simulink model "Michaels_CVModel_fast8"  (R2020a)
settings: Solver=ode23  StartTime=0.0  StopTime=30  RelTol=1e-2  EnableMultiTasking=on
model workspace (MAT data in the model file):
  Eao = 1.88
  Eesla = 0.58
  Eeslvf = 5.2
  Eesra = 0.63
  Eesrvf = 1.75
  Emaxspt = 48.75
  Epa = 0.15
  Epu = 0.04
  Esa = 0.37
  Esv = 0.013
  Evc = 0.03
  GpLV = 0
  GpRR = 11
  GpRV = 0
  GpRsa = 0
  GpV0 = 0
  GsLV = 0.007
  GsRR = 11
  GsRV = 0.022
  GsRsa = -0.05
  GsV0 = 31
  Ka = 4.4
  Lao = 0.0022
  Lav = 0.000354
  Lmt = 7.697e-05
  Lpa = 7.697e-05
  Lpv = 0.0001043
  Ltc = 8.009e-05
  P0la = 0.5
  P0lvf = 0.98
  P0pcd = 0.5
  P0ra = 0.5
  P0rvf = 0.91
  P0spt = 0.46
  PV : AO (value not decoded)
  PVao = [327.9; 100.9]
  Rao = 0.28
  Rav = 0.02
  Rla2pu = 0.5
  Rmt = 0.01
  Rpa = 0.12
  Rpa_Vals = 0.12
  Rpu = 0.006
  Rpv = 0.02
  Rra = 0.012
  Rsa = 0.74
  Rsv = 0.12
  Rtc = 0.01
  Tc = 1
  Tsys0 = 0.6
  V0la = 30
  V0lvf = 45
  V0pcd = 200
  V0ra = 25
  V0rvf = 50
  V0spt = 10
  Vdla = 15
  Vdlvf = 16
  Vdra = 15
  Vdrvf = 40
  Vdspt = 10
  Vlv0 = 100
  Vperi = 51
  Vrv0 = 105
  Vuao = 260.8
  Vupa = 91
  Vupu = 132
  Vusa = 287.4
  Vusv = 1976.1
  Vuvc = 136.17
  amin = -2
  artBrLVcontConti = []
  artBrLVcontDigi = [0 0 0 0 0 0 0 0 0 0 0 0 ... (240 elements, 1x240)]
  artBrRRConti = []
  artBrRRDigi = [0 0 0 0 0 0 0 0 0 0 1.57142857143 3.14285714286 ... (240 elements, 1x240)]
  artBrRVcontConti = []
  artBrRVcontDigi = [0 0 0 0 0 0 0 0 0 0 0 0 ... (240 elements, 1x240)]
  artBrRsaConti = []
  artBrRsaDigi = [0 0 0 0 0 0 0 0 0 0 0 0 ... (480 elements, 1x480)]
  artBrV0Conti = []
  artBrV0Digi = [0 0 0 0 0 0 0 0 0 0 0 0 ... (640 elements, 1x640)]
  atriumA = 1
  baroSampFreq = 16
  cP0la = 0.5
  cP0lvf = 0.98
  cP0ra = 0.5
  cP0rvf = 0.91
  cT = 1
  cVtotal = 5400
  clambdala = 0.13
  clambdalvf = 0.028
  clambdara = 0.13
  clambdarvf = 0.028
  deac = 0.0004
  ksys = 0.075
  lambdala = 0.065
  lambdalvf = 0.042
  lambdapcd = 0.005
  lambdara = 0.065
  lambdarvf = 0.028
  lambdaspt = 0.4
  pThor = 0
  params : object (value not decoded)
  sampleTime = 0.005
  svcPressureChange_MCS = 0
  svrMult = 1
  tStepOn = 1000000000
  t_baroOn = 1000000
  t_testBed_start = 1000000
  venk1 = 0.5
  venk2 = 0.5
symbols that are objects in the model workspace (value not decoded): PV
undefined symbols (not defined in the file): dfilt
libraries: simulink x85, fl_lib x39, nesl_utility x24, cstblocks x9, dspstat3 x9, dspobslib x5, SimscapeFluids_lib x5, sh_lib x1
(part 5 of 5)

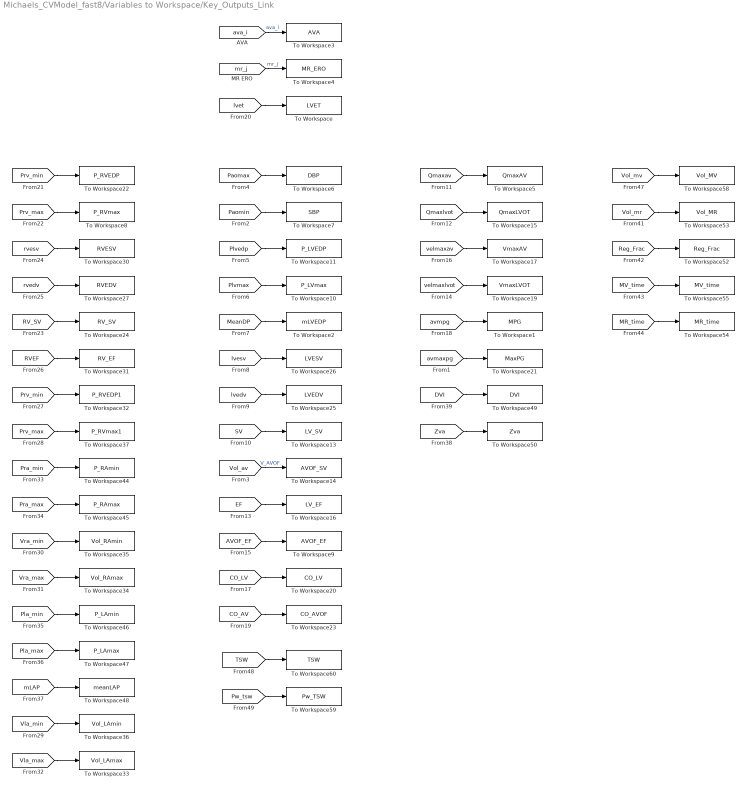
== system Michaels_CVModel_fast8/Variables to Workspace/Key_Outputs_Link ==
  To Workspace : ToWorkspace  VariableName=LVET  SampleTime=0.005
      settings: MaxDataPoints=1
  To Workspace1 : ToWorkspace  VariableName=MPG  SampleTime=0.01
      settings: MaxDataPoints=1
  To Workspace10 : ToWorkspace  VariableName=P_LVmax  SampleTime=0.01
      settings: MaxDataPoints=1
  To Workspace11 : ToWorkspace  VariableName=P_LVEDP  SampleTime=0.01
      settings: MaxDataPoints=1
  To Workspace13 : ToWorkspace  VariableName=LV_SV  SampleTime=0.01
      settings: MaxDataPoints=1
  To Workspace14 : ToWorkspace  VariableName=AVOF_SV  SampleTime=0.01
      settings: MaxDataPoints=1
  To Workspace15 : ToWorkspace  VariableName=QmaxLVOT  SampleTime=0.01
      settings: MaxDataPoints=1
  To Workspace16 : ToWorkspace  VariableName=LV_EF  SampleTime=0.01
      settings: MaxDataPoints=1
  To Workspace17 : ToWorkspace  VariableName=VmaxAV  SampleTime=0.01
      settings: MaxDataPoints=1
  To Workspace19 : ToWorkspace  VariableName=VmaxLVOT  SampleTime=0.01
      settings: MaxDataPoints=1
  To Workspace2 : ToWorkspace  VariableName=mLVEDP  SampleTime=0.01
      settings: MaxDataPoints=1
  To Workspace20 : ToWorkspace  VariableName=CO_LV  SampleTime=0.01
      settings: MaxDataPoints=1
  To Workspace21 : ToWorkspace  VariableName=MaxPG  SampleTime=0.01
      settings: MaxDataPoints=1
  To Workspace22 : ToWorkspace  VariableName=P_RVEDP  SampleTime=0.01
      settings: MaxDataPoints=1
  To Workspace23 : ToWorkspace  VariableName=CO_AVOF  SampleTime=0.01
      settings: MaxDataPoints=1
  To Workspace24 : ToWorkspace  VariableName=RV_SV  SampleTime=0.01
      settings: MaxDataPoints=1
  To Workspace25 : ToWorkspace  VariableName=LVEDV  SampleTime=0.01
      settings: MaxDataPoints=1
  To Workspace26 : ToWorkspace  VariableName=LVESV  SampleTime=0.01
      settings: MaxDataPoints=1
  To Workspace27 : ToWorkspace  VariableName=RVEDV  SampleTime=0.01
      settings: MaxDataPoints=1
  To Workspace3 : ToWorkspace  VariableName=AVA  SampleTime=0.005
      settings: MaxDataPoints=1
  To Workspace30 : ToWorkspace  VariableName=RVESV  SampleTime=0.01
      settings: MaxDataPoints=1
  To Workspace31 : ToWorkspace  VariableName=RV_EF  SampleTime=0.01
      settings: MaxDataPoints=1
  To Workspace32 : ToWorkspace  VariableName=P_RVEDP1  SampleTime=0.01
      settings: MaxDataPoints=1
  To Workspace33 : ToWorkspace  VariableName=Vol_LAmax  SampleTime=0.01
      settings: MaxDataPoints=1
  To Workspace34 : ToWorkspace  VariableName=Vol_RAmax  SampleTime=0.01
      settings: MaxDataPoints=1
  To Workspace35 : ToWorkspace  VariableName=Vol_RAmin  SampleTime=0.01
      settings: MaxDataPoints=1
  To Workspace36 : ToWorkspace  VariableName=Vol_LAmin  SampleTime=0.01
      settings: MaxDataPoints=1
  To Workspace37 : ToWorkspace  VariableName=P_RVmax1  SampleTime=0.01
      settings: MaxDataPoints=1
  To Workspace4 : ToWorkspace  VariableName=MR_ERO  SampleTime=0.005
      settings: MaxDataPoints=1
  To Workspace44 : ToWorkspace  VariableName=P_RAmin  SampleTime=0.01
      settings: MaxDataPoints=1
  To Workspace45 : ToWorkspace  VariableName=P_RAmax  SampleTime=0.01
      settings: MaxDataPoints=1
  To Workspace46 : ToWorkspace  VariableName=P_LAmin  SampleTime=0.01
      settings: MaxDataPoints=1
  To Workspace47 : ToWorkspace  VariableName=P_LAmax  SampleTime=0.01
      settings: MaxDataPoints=1
  To Workspace48 : ToWorkspace  VariableName=meanLAP  SampleTime=0.01
      settings: MaxDataPoints=1
  To Workspace49 : ToWorkspace  VariableName=DVI  SampleTime=0.01
      settings: MaxDataPoints=1
  To Workspace5 : ToWorkspace  VariableName=QmaxAV  SampleTime=0.01
      settings: MaxDataPoints=1
  To Workspace50 : ToWorkspace  VariableName=Zva  SampleTime=0.01
      settings: MaxDataPoints=1
  To Workspace52 : ToWorkspace  VariableName=Reg_Frac  SampleTime=0.01
      settings: MaxDataPoints=1
  To Workspace53 : ToWorkspace  VariableName=Vol_MR  SampleTime=0.01
      settings: MaxDataPoints=1
  To Workspace54 : ToWorkspace  VariableName=MR_time  SampleTime=0.01
      settings: MaxDataPoints=1
  To Workspace55 : ToWorkspace  VariableName=MV_time  SampleTime=0.01
      settings: MaxDataPoints=1
  To Workspace58 : ToWorkspace  VariableName=Vol_MV  SampleTime=0.01
      settings: MaxDataPoints=1
  To Workspace59 : ToWorkspace  VariableName=Pw_TSW  SampleTime=0.01
      settings: MaxDataPoints=1
  To Workspace6 : ToWorkspace  VariableName=DBP  SampleTime=0.01
      settings: MaxDataPoints=1
  To Workspace60 : ToWorkspace  VariableName=TSW  SampleTime=0.01
      settings: MaxDataPoints=1
  To Workspace7 : ToWorkspace  VariableName=SBP  SampleTime=0.01
      settings: MaxDataPoints=1
  To Workspace8 : ToWorkspace  VariableName=P_RVmax  SampleTime=0.01
      settings: MaxDataPoints=1
  To Workspace9 : ToWorkspace  VariableName=AVOF_EF  SampleTime=0.01
      settings: MaxDataPoints=1
  wires:
  [ava_i] -> To Workspace3/1  "ava_i"
  [mr_j] -> To Workspace4/1  "mr_j"
  [Paomax] -> To Workspace6/1
  [Paomin] -> To Workspace7/1
  [Plvedp] -> To Workspace11/1
  [Plvmax] -> To Workspace10/1
  [MeanDP] -> To Workspace2/1
  [lvedv] -> To Workspace25/1
  [lvesv] -> To Workspace26/1
  [SV] -> To Workspace13/1
  [Vol_av] -> To Workspace14/1  "V_AVOF"
  [Qmaxav] -> To Workspace5/1
  [Qmaxlvot] -> To Workspace15/1
  [EF] -> To Workspace16/1
  [velmaxlvot] -> To Workspace19/1
  [velmaxav] -> To Workspace17/1
  [avmpg] -> To Workspace1/1
  [avmaxpg] -> To Workspace21/1
  [CO_LV] -> To Workspace20/1
  [CO_AV] -> To Workspace23/1
  [lvet] -> To Workspace/1
  [rvesv] -> To Workspace30/1
  [rvedv] -> To Workspace27/1
  [Prv_max] -> To Workspace8/1
  [Prv_min] -> To Workspace22/1
  [RVEF] -> To Workspace31/1
  [RV_SV] -> To Workspace24/1
  [Prv_min] -> To Workspace32/1
  [Prv_max] -> To Workspace37/1
  [Vra_min] -> To Workspace35/1
  [Pra_min] -> To Workspace44/1
  [Pra_max] -> To Workspace45/1
  [Vra_max] -> To Workspace34/1
  [Vla_max] -> To Workspace33/1
  [Pla_max] -> To Workspace47/1
  [Pla_min] -> To Workspace46/1
  [Vla_min] -> To Workspace36/1
  [mLAP] -> To Workspace48/1
  [Zva] -> To Workspace50/1
  [DVI] -> To Workspace49/1
  [Vol_mr] -> To Workspace53/1
  [Reg_Frac] -> To Workspace52/1
  [MR_time] -> To Workspace54/1
  [MV_time] -> To Workspace55/1
  [Vol_mv] -> To Workspace58/1
  [Pw_tsw] -> To Workspace59/1
  [TSW] -> To Workspace60/1
  [AVOF_EF] -> To Workspace9/1

== system Michaels_CVModel_fast8/Variables to Workspace/Pressure ==
  From1 : From  Commented=on  GotoTag=Pthor2  TagVisibility=global
      settings: CloseFcn=tagdialog Close
  From44 : From  Commented=on  GotoTag=Prv  TagVisibility=global
      settings: CloseFcn=tagdialog Close
  From45 : From  Commented=on  GotoTag=Pla  TagVisibility=global
      settings: CloseFcn=tagdialog Close
  From46 : From  Commented=on  GotoTag=Pra  TagVisibility=global
      settings: CloseFcn=tagdialog Close
  From47 : From  Commented=on  GotoTag=Ppa  TagVisibility=global
      settings: CloseFcn=tagdialog Close
  From48 : From  Commented=on  GotoTag=Ppu  TagVisibility=global
      settings: CloseFcn=tagdialog Close
  From49 : From  Commented=on  GotoTag=Psa  TagVisibility=global
      settings: CloseFcn=tagdialog Close
  From50 : From  Commented=on  GotoTag=Psv  TagVisibility=global
      settings: CloseFcn=tagdialog Close
  From51 : From  Commented=on  GotoTag=Pao  TagVisibility=global
      settings: CloseFcn=tagdialog Close
  From52 : From  Commented=on  GotoTag=Pvc  TagVisibility=global
      settings: CloseFcn=tagdialog Close
  From53 : From  Commented=on  GotoTag=Pthor  TagVisibility=global
      settings: CloseFcn=tagdialog Close
  To Workspace1 : ToWorkspace  VariableName=P_LV  SampleTime=0.005
      settings: MaxDataPoints=201
  To Workspace10 : ToWorkspace  Commented=on  VariableName=P_THOR  SampleTime=0.005
  To Workspace11 : ToWorkspace  Commented=on  VariableName=P_VC  SampleTime=0.005
  To Workspace12 : ToWorkspace  Commented=on  VariableName=P_THOR2  SampleTime=0.005
  To Workspace13 : ToWorkspace  VariableName=P_LV2  SampleTime=0.005
      settings: MaxDataPoints=201
  To Workspace2 : ToWorkspace  Commented=on  VariableName=P_RV  SampleTime=0.005
  To Workspace3 : ToWorkspace  Commented=on  VariableName=P_LA  SampleTime=0.005
  To Workspace4 : ToWorkspace  Commented=on  VariableName=P_RA  SampleTime=0.005
  To Workspace5 : ToWorkspace  Commented=on  VariableName=P_SA  SampleTime=0.005
  To Workspace6 : ToWorkspace  Commented=on  VariableName=P_AO  SampleTime=0.005
  To Workspace7 : ToWorkspace  Commented=on  VariableName=P_SV  SampleTime=0.005
  To Workspace8 : ToWorkspace  Commented=on  VariableName=P_PA  SampleTime=0.005
  To Workspace9 : ToWorkspace  Commented=on  VariableName=P_PU  SampleTime=0.005
  wires:
  [Plv] -> To Workspace1/1  "P_LV"
  From44/1 -> To Workspace2/1  "P_RV"
  From45/1 -> To Workspace3/1  "P_LA"
  From46/1 -> To Workspace4/1  "P_RA"
  From49/1 -> To Workspace5/1  "P_SA"
  From51/1 -> To Workspace6/1  "P_AO"
  From50/1 -> To Workspace7/1  "P_SV"
  From47/1 -> To Workspace8/1  "P_PA"
  From48/1 -> To Workspace9/1  "P_PU"
  From53/1 -> To Workspace10/1  "P_THOR"
  From52/1 -> To Workspace11/1  "P_VC"
  From1/1 -> To Workspace12/1
  [PLV_SSc] -> To Workspace13/1

== system Michaels_CVModel_fast8/Variables to Workspace/Settings ==
  01Constant42 : Constant  Value=Eeslvf
  02Constant46 : Constant  Value=Eesrvf
  03Constant28 : Constant  Value=Eesla
  04Constant38 : Constant  Value=Eesra
  101Constant1 : Constant  Value=Eao
  101Constant2 : Constant  Value=Rao
  10Constant1 : Constant  Value=Vusa
  10Constant2 : Constant  Value=Rpu
  10Constant43 : Constant  Value=Vdlvf
  11Constant1 : Constant  Value=Vuao
  11Constant2 : Constant  Value=Lao
  11Constant41 : Constant  Value=V0lvf
  12Constant47 : Constant  Value=Vdrvf
  13Constant45 : Constant  Value=V0rvf
  14Constant29 : Constant  Value=Vdla
  15Constant27 : Constant  Value=V0la
  16Constant39 : Constant  Value=Vdra
  17Constant37 : Constant  Value=V0ra
  18Constant30 : Constant  Value=V0pcd
  20Constant34 : Constant  Value=lambdalvf
  21Constant35 : Constant  Value=lambdarvf
  22Constant32 : Constant  Value=lambdala
  23Constant33 : Constant  Value=lambdara
  24Constant36 : Constant  Value=lambdapcd
  5Constant44 : Constant  Value=P0lvf
  6Constant48 : Constant  Value=P0rvf
  7Constant31 : Constant  Value=P0la
  8Constant40 : Constant  Value=P0ra
  9Constant49 : Constant  Value=P0pcd
  Mux1 : Mux  Inputs=18
  Mux2 : Mux  Inputs=8
  Mux3 : Mux  Inputs=6
  Rla2pu : Constant  Value=Rla2pu
  Settings : Scope  Commented=on  NumInputPorts=2
  Settings1 : Scope  Commented=on
  wires:
  18Constant30/1 -> Mux1/18  "V0pcd"
  9Constant49/1 -> Mux1/17  "P0pcd"
  8Constant40/1 -> Mux1/16  "P0ra"
  16Constant39/1 -> Mux1/15  "Vdra"
  17Constant37/1 -> Mux1/14  "V0ra"
  04Constant38/1 -> Mux1/13  "Eesra"
  7Constant31/1 -> Mux1/12  "P0la"
  14Constant29/1 -> Mux1/11  "Vdla"
  15Constant27/1 -> Mux1/10  "V0la"
  03Constant28/1 -> Mux1/9  "Eesla"
  6Constant48/1 -> Mux1/8  "P0rvf"
  12Constant47/1 -> Mux1/7  "Vdrvf"
  13Constant45/1 -> Mux1/6  "V0rvf"
  02Constant46/1 -> Mux1/5  "Eesrvf"
  5Constant44/1 -> Mux1/4  "P0lvf"
  10Constant43/1 -> Mux1/3  "Vdlvf"
  11Constant41/1 -> Mux1/2  "V0lvf"
  01Constant42/1 -> Mux1/1  "Eeslvf"
  22Constant32/1 -> Mux2/1  "lambdala"
  23Constant33/1 -> Mux2/2  "lambdara"
  20Constant34/1 -> Mux2/3  "lambdalvf"
  21Constant35/1 -> Mux2/4  "lambdarvf"
  24Constant36/1 -> Mux2/5  "lambdapcd"
  Mux1/1 -> Settings/1
  Mux2/1 -> Settings/2
  [Rsa] -> Mux2/6  "xRsa"
  [Vusv] -> Mux2/7  "xVusv"
  Rla2pu/1 -> Mux2/8  "xRla2Pu"
  11Constant1/1 -> Mux3/2  "Vuao"
  101Constant1/1 -> Mux3/1  "Eesao"
  10Constant1/1 -> Mux3/3  "Vusa"
  101Constant2/1 -> Mux3/4  "Rao"
  11Constant2/1 -> Mux3/5  "Lao"
  10Constant2/1 -> Mux3/6  "Rpu"
  Mux3/1 -> Settings1/1

== system Michaels_CVModel_fast8/Variables to Workspace/Volume ==
  From1 : From  Commented=on  GotoTag=AVOF_Vol  TagVisibility=global
      settings: CloseFcn=tagdialog Close
  From54 : From  Commented=on  GotoTag=Vlv  TagVisibility=global
      settings: CloseFcn=tagdialog Close
  From55 : From  Commented=on  GotoTag=Vrv  TagVisibility=global
      settings: CloseFcn=tagdialog Close
  From56 : From  Commented=on  GotoTag=Vla  TagVisibility=global
      settings: CloseFcn=tagdialog Close
  From57 : From  Commented=on  GotoTag=Vra  TagVisibility=global
      settings: CloseFcn=tagdialog Close
  From58 : From  Commented=on  GotoTag=Vsv  TagVisibility=global
      settings: CloseFcn=tagdialog Close
  From59 : From  Commented=on  GotoTag=Vsa  TagVisibility=global
      settings: CloseFcn=tagdialog Close
  From60 : From  Commented=on  GotoTag=Vpa  TagVisibility=global
      settings: CloseFcn=tagdialog Close
  From61 : From  Commented=on  GotoTag=Vpu  TagVisibility=global
      settings: CloseFcn=tagdialog Close
  From62 : From  Commented=on  GotoTag=Vspt  TagVisibility=global
      settings: CloseFcn=tagdialog Close
  From63 : From  Commented=on  GotoTag=Vvc  TagVisibility=global
      settings: CloseFcn=tagdialog Close
  From64 : From  Commented=on  GotoTag=Vao  TagVisibility=global
      settings: CloseFcn=tagdialog Close
  To Workspace1 : ToWorkspace  Commented=on  VariableName=V_AV  SampleTime=0.005
      settings: MaxDataPoints=201
  To Workspace13 : ToWorkspace  VariableName=V_Total  SampleTime=0.005
  To Workspace14 : ToWorkspace  Commented=on  VariableName=V_VC  SampleTime=0.005
  To Workspace15 : ToWorkspace  Commented=on  VariableName=V_RV  SampleTime=0.005
  To Workspace16 : ToWorkspace  Commented=on  VariableName=V_LA  SampleTime=0.005
  To Workspace17 : ToWorkspace  Commented=on  VariableName=V_RA  SampleTime=0.005
  To Workspace18 : ToWorkspace  Commented=on  VariableName=V_SA  SampleTime=0.005
  To Workspace19 : ToWorkspace  Commented=on  VariableName=V_AO  SampleTime=0.005
  To Workspace2 : ToWorkspace  Commented=on  VariableName=V_LV  SampleTime=0.005
      settings: MaxDataPoints=201  Save2DSignal=2-D array (concatenate along first dimension)
  To Workspace20 : ToWorkspace  Commented=on  VariableName=V_SV  SampleTime=0.005
  To Workspace21 : ToWorkspace  Commented=on  VariableName=V_PA  SampleTime=0.005
  To Workspace23 : ToWorkspace  Commented=on  VariableName=V_spt  SampleTime=0.005
  To Workspace24 : ToWorkspace  Commented=on  VariableName=V_PU  SampleTime=0.005
  wires:
  From54/1 -> To Workspace2/1  "V_LV"
  From55/1 -> To Workspace15/1  "V_RV"
  From56/1 -> To Workspace16/1  "V_LA"
  From57/1 -> To Workspace17/1  "V_RA"
  From62/1 -> To Workspace23/1  "V_SPT"
  [Vtotal] -> To Workspace13/1  "V_Total"
  From63/1 -> To Workspace14/1  "V_VC"
  From59/1 -> To Workspace18/1  "V_SA"
  From64/1 -> To Workspace19/1  "V_AO"
  From58/1 -> To Workspace20/1  "V_SV"
  From60/1 -> To Workspace21/1  "V_PA"
  From61/1 -> To Workspace24/1  "V_PU"
  From1/1 -> To Workspace1/1  "V_AVOF"

== system Michaels_CVModel_fast8/ev/Activation - Atria ==
  note: Activation Functions - atria
  Action 1 - Sin Squared : Subsystem  TreatAsAtomicUnit=on
  Action 2 - cos Squared1 : Subsystem  TreatAsAtomicUnit=on
  Condition 1 : Subsystem
  Condition 2 : Subsystem
  Else - 0 : Subsystem  TreatAsAtomicUnit=on
  If : If  NumInputs=2  IfExpression=u1 == 1  ElseIfExpressions=u2 == 1
  Mux : Mux  Inputs=3
  Mux1 : Mux
  Mux2 : Mux  Commented=on  Inputs=2
  Scope2 : Scope  Commented=on
  ea : Merge  Inputs=3
  Out1 : Outport
  wires:
  Condition 1/1(Out1) -> If/1, Mux2/1
  Condition 2/1(Out1) -> If/2, Mux2/2
  If/3 -> Else - 0/Action
  Else - 0/1(Out1) -> ea/3
  [Tsh_a] -> Mux/2, Mux1/2
  [t] -> Mux/1, Mux1/1
  [Tr_A] -> Mux/3, Mux1/3
  Mux/1 -> Action 1 - Sin Squared/1(In1)
  If/1 -> Action 1 - Sin Squared/Action
  Mux1/1 -> Action 2 - cos Squared1/1(In1)
  If/2 -> Action 2 - cos Squared1/Action
  [TsysA] -> Mux1/4
  Action 1 - Sin Squared/1(Out1) -> ea/1
  Action 2 - cos Squared1/1(Out1) -> ea/2
  Mux2/1 -> Scope2/1
  ea/1 -> Out1/1

== system Michaels_CVModel_fast8/ev/Activation - Ventricle ==
  note: Activation Functions - Ventricle
  Action 1 - Sin Squared : Subsystem  TreatAsAtomicUnit=on
  Action 2 - cos Squared1 : Subsystem  TreatAsAtomicUnit=on
  Condition 1 : Subsystem
  Condition 2 : Subsystem
  Else - 0 : Subsystem  TreatAsAtomicUnit=on
  If : If  NumInputs=2  IfExpression=u1 == 1  ElseIfExpressions=u2 == 1
  Mux : Mux  Inputs=3
  Mux1 : Mux
  Mux2 : Mux  Commented=on  Inputs=2
  Scope2 : Scope  Commented=on
  ev : Merge  Inputs=3
  1 : Outport
  wires:
  Condition 1/1(Out1) -> If/1, Mux2/1
  Condition 2/1(Out1) -> If/2, Mux2/2
  If/3 -> Else - 0/Action
  Else - 0/1(Out1) -> ev/3
  [Tsh_v] -> Mux/2, Mux1/2
  [t] -> Mux/1, Mux1/1
  [Tr_V] -> Mux/3, Mux1/3
  Mux/1 -> Action 1 - Sin Squared/1(In1)
  If/1 -> Action 1 - Sin Squared/Action
  Mux1/1 -> Action 2 - cos Squared1/1(In1)
  If/2 -> Action 2 - cos Squared1/Action
  [TsysV] -> Mux1/4
  Action 1 - Sin Squared/1(Out1) -> ev/1
  Action 2 - cos Squared1/1(Out1) -> ev/2
  Mux2/1 -> Scope2/1
  ev/1 -> 1/1

== system Michaels_CVModel_fast8/ev/Activation - Ventricle_half ==
  note: Activation Functions - Ventricle
  Action 1 - Sin Squared : Subsystem  TreatAsAtomicUnit=on
  Action 2 - cos Squared1 : Subsystem  TreatAsAtomicUnit=on
  Condition 1 : Subsystem
  Condition 2 : Subsystem
  Else - 0 : Subsystem  TreatAsAtomicUnit=on
  If : If  NumInputs=2  IfExpression=u1 == 1  ElseIfExpressions=u2 == 1
  Mux : Mux  Inputs=3
  Mux1 : Mux
  Mux2 : Mux  Commented=on  Inputs=2
  Scope2 : Scope  Commented=on
  ev : Merge  Inputs=3
  evcos : Outport
  wires:
  Condition 1/1(Out1) -> If/1, Mux2/1
  Condition 2/1(Out1) -> If/2, Mux2/2
  If/3 -> Else - 0/Action
  Else - 0/1(Out1) -> ev/3
  [Tsh_v] -> Mux/2, Mux1/2
  [t] -> Mux/1, Mux1/1
  [Tr_V] -> Mux/3, Mux1/3
  Mux/1 -> Action 1 - Sin Squared/1(In1)
  If/1 -> Action 1 - Sin Squared/Action
  Mux1/1 -> Action 2 - cos Squared1/1(In1)
  If/2 -> Action 2 - cos Squared1/Action
  [TsysV] -> Mux1/4
  Action 1 - Sin Squared/1(Out1) -> ev/1
  Action 2 - cos Squared1/1(Out1) -> ev/2
  Mux2/1 -> Scope2/1
  ev/1 -> evcos/1

== system Michaels_CVModel_fast8/ev/Ev off-set ==
  note: Offset to reduce delay btw LV response to activation
  Inport : Inport
  Add : Sum  Inputs=+-
  Constant : Constant  Value=0.001
  Gain2 : Gain  Gain=1.001
  Saturation : Saturate  UpperLimit=inf  LowerLimit=0
  " " : Outport
  wires:
  Gain2/1 -> Add/1
  Add/1 -> Saturation/1
  Constant/1 -> Add/2
  Inport/1 -> Gain2/1
  Saturation/1 -> " "/1

== system Michaels_CVModel_fast8/Baroreflex/Baroreflex Heldt/avg filter ==
  Raw : Inport
  Buffer : Buffer  N=1.5*1/0.01  V=1.5*1/0.01-1
  Fcn : Fcn  Expr=(u(1)+u(2))/2
  MinMax : MinMax
  MinMax1 : MinMax  Function=max
  Mux : Mux  Inputs=2
  Mux1 : Mux  Commented=on
  SH 0.01 : ZeroOrderHold  SampleTime=0.01
  Scope : Scope  Commented=on
  Unbuffer : Unbuffer
  Unbuffer1 : Unbuffer
  Avg : Outport
  wires:
  Raw/1 -> SH 0.01/1, Mux1/4
  SH 0.01/1 -> Buffer/1
  Buffer/1 -> MinMax/1, MinMax1/1
  MinMax1/1 -> Unbuffer/1
  Mux/1 -> Fcn/1
  Unbuffer/1 -> Mux/2, Mux1/2
  MinMax/1 -> Unbuffer1/1
  Unbuffer1/1 -> Mux/1, Mux1/1
  Fcn/1 -> Avg/1, Mux1/3
  Mux1/1 -> Scope/1

== system Michaels_CVModel_fast8/Baroreflex/Baroreflex Heldt/sigmoid limit ==
  In1 : Inport
  Gain : Gain  Gain=1/18
  Gain1 : Gain  Gain=18
  Trigonometric Function : Trigonometry  Operator=atan
  Out1 : Outport
  wires:
  Gain/1 -> Trigonometric Function/1
  Trigonometric Function/1 -> Gain1/1
  In1/1 -> Gain/1
  Gain1/1 -> Out1/1

== system Michaels_CVModel_fast8/Baroreflex/Baroreflex Heldt cont/Filter ==
  Raw : Inport
  Buffer : Buffer  N=1.5*1/0.01  V=1.5*1/0.01-1
  Fcn : Fcn  Expr=(1*u(1)+1*u(2))/2
  MinMax : MinMax  Function=max
  MinMax1 : MinMax
  Mux : Mux  Inputs=2
  Mux1 : Mux
  SH 0.01 : ZeroOrderHold  SampleTime=0.01
  Scope : Scope  Commented=on
  Unbuffer : Unbuffer
  Unbuffer1 : Unbuffer
  Filtered : Outport
  wires:
  Raw/1 -> SH 0.01/1, Mux1/4
  SH 0.01/1 -> Buffer/1
  Buffer/1 -> MinMax/1, MinMax1/1
  MinMax1/1 -> Unbuffer/1
  Mux/1 -> Fcn/1
  Unbuffer/1 -> Mux/2, Mux1/2
  MinMax/1 -> Unbuffer1/1
  Unbuffer1/1 -> Mux/1, Mux1/1
  Fcn/1 -> Filtered/1, Mux1/3
  Mux1/1 -> Scope/1

== system Michaels_CVModel_fast8/Baroreflex/Baroreflex Heldt cont/sigmoid limit ==
  In1 : Inport
  Gain : Gain  Gain=1/18
  Gain1 : Gain  Gain=18
  Trigonometric Function : Trigonometry  Operator=atan
  Out1 : Outport
  wires:
  Gain/1 -> Trigonometric Function/1
  Trigonometric Function/1 -> Gain1/1
  In1/1 -> Gain/1
  Gain1/1 -> Out1/1

== system Michaels_CVModel_fast8/Graphs and Scopes/SW Scrap/Stroke Work Action ==
  In1 : Inport
  Inport2 : Inport  Port=2
  Action Port : ActionPort
  Integrator1 : Integrator  ExternalReset=rising
  Integrator2 : Integrator  ExternalReset=rising
  Integrator3 : Integrator  ExternalReset=rising
  Product : Product
  Scope : Scope  NumInputPorts=2
  Outport : Outport
  wires:
  Integrator1/1 -> Scope/1, Outport/1
  Product/1 -> Integrator1/1
  Inport2/1 -> Product/2, Scope/2, Integrator1/2
  In1/1 -> Product/1

== system Michaels_CVModel_fast8/Graphs and Scopes/SW Scrap/Stroke Work Action1 ==
  In1 : Inport
  Inport2 : Inport  Port=2
  Action Port : ActionPort
  Integrator2 : Integrator  ExternalReset=rising
  Integrator3 : Integrator  ExternalReset=rising
  Product : Product
  Scope : Scope  NumInputPorts=2
  Outport : Outport
  wires:
  In1/1 -> Product/1
  Inport2/1 -> Scope/2, Product/2
  Product/1 -> Scope/1, Outport/1

== system Michaels_CVModel_fast8/Graphs and Scopes/SW Scrap/Stroke Work Action2 ==
  In1 : Inport
  In2 : Inport  Port=2
  Inport2 : Inport  Port=3
  Action Port : ActionPort  InitializeStates=reset
  Integrator1 : Integrator  ExternalReset=either
  Product : Product
  Scope : Scope  NumInputPorts=2
  Outport : Outport
  wires:
  In1/1 -> Product/1
  Inport2/1 -> Product/2
  Product/1 -> Integrator1/1
  Integrator1/1 -> Outport/1, Scope/1
  In2/1 -> Integrator1/2

== system Michaels_CVModel_fast8/Graphs and Scopes/SW Scrap/Stroke Work Action3 ==
  In1 : Inport
  Inport2 : Inport  Port=2
  Action Port : ActionPort  InitializeStates=reset
  Integrator : Integrator  ExternalReset=either
  Product : Product
  Scope : Scope  NumInputPorts=2
  Outport : Outport
  wires:
  Product/1 -> Integrator/1
  Inport2/1 -> Product/2, Scope/2
  In1/1 -> Integrator/2, Product/1
  Integrator/1 -> Outport/1, Scope/1

== system Michaels_CVModel_fast8/Graphs and Scopes/SW Scrap/Stroke Work Action5 ==
  In1 : Inport
  Inport2 : Inport  Port=2
  Action Port : ActionPort
  Integrator1 : Integrator  ExternalReset=rising
  Product : Product
  Scope : Scope  NumInputPorts=2
  Outport : Outport
  wires:
  Integrator1/1 -> Scope/1, Outport/1
  Product/1 -> Integrator1/1
  Inport2/1 -> Integrator1/2, Product/2
  In1/1 -> Product/1

== system Michaels_CVModel_fast8/Graphs and Scopes/SW Scrap/Stroke Work Action6 ==
  In1 : Inport
  Inport2 : Inport  Port=2
  Action Port : ActionPort
  Integrator : Integrator  ExternalReset=rising
  Product : Product
  Scope : Scope  NumInputPorts=2
  Outport : Outport
  wires:
  Integrator/1 -> Scope/1, Outport/1
  In1/1 -> Integrator/2, Product/1
  Inport2/1 -> Scope/2, Product/2
  Product/1 -> Integrator/1

== system Michaels_CVModel_fast8/Graphs and Scopes/SW Scrap/Triggered Subsystem ==
  Outport : Inport
  Trigger : TriggerPort  VariantControl=(inherit)
  SW Q_AV1 : Outport  VectorParamsAs1DForOutWhenUnconnected=off
  wires:
  Outport/1 -> SW Q_AV1/1  "SW"

== system Michaels_CVModel_fast8/Graphs and Scopes/SW Scrap/Triggered Subsystem1 ==
  Outport : Inport
  Trigger : TriggerPort  VariantControl=(inherit)
  SW Q_AV1 : Outport  VectorParamsAs1DForOutWhenUnconnected=off
  wires:
  Outport/1 -> SW Q_AV1/1  "SW"

== system Michaels_CVModel_fast8/Graphs and Scopes/SW Scrap/Triggered Subsystem3 ==
  Outport : Inport
  Trigger : TriggerPort  VariantControl=(inherit)
  SW Q_AV1 : Outport  VectorParamsAs1DForOutWhenUnconnected=off
  wires:
  Outport/1 -> SW Q_AV1/1  "SW"

== system Michaels_CVModel_fast8/Stroke Work Calcs/Stroke Work Calc AVOF/Triggered Subsystem ==
  In1 : Inport
  In2 : Inport  Port=2
  Trigger : TriggerPort  TriggerType=falling  VariantControl=(inherit)
  Out1 : Outport  VectorParamsAs1DForOutWhenUnconnected=off
  Out2 : Outport  Port=2  VectorParamsAs1DForOutWhenUnconnected=off
  wires:
  In2/1 -> Out2/1  "SW"
  In1/1 -> Out1/1  "Energy"

== system Michaels_CVModel_fast8/Stroke Work Calcs/Stroke Work MR_Vol/Triggered Subsystem ==
  In1 : Inport
  In2 : Inport  Port=2
  Trigger : TriggerPort  TriggerType=falling  VariantControl=(inherit)
  Out1 : Outport  VectorParamsAs1DForOutWhenUnconnected=off
  Out2 : Outport  Port=2  VectorParamsAs1DForOutWhenUnconnected=off
  wires:
  In2/1 -> Out2/1  "SW"
  In1/1 -> Out1/1  "Energy"

== system Michaels_CVModel_fast8/Stroke Work Calcs/Stroke Work Q_AV/Stroke Work Action ==
  In1 : Inport
  In2 : Inport  Port=2
  Inport2 : Inport  Port=3
  Action Port : ActionPort  InitializeStates=reset  ActionPortLabel=if(u1 == 1)
  Integrator1 : Integrator  ExternalReset=rising
  Product : Product
  Scope : Scope  Commented=on  NumInputPorts=2
  Outport : Outport
  wires:
  In2/1 -> Integrator1/2
  In1/1 -> Product/1
  Inport2/1 -> Product/2, Scope/2
  Product/1 -> Integrator1/1
  Integrator1/1 -> Outport/1, Scope/1

== system Michaels_CVModel_fast8/Stroke Work Calcs/Stroke Work Q_AV/Triggered Subsystem1 ==
  Outport : Inport
  Trigger : TriggerPort  TriggerType=falling  VariantControl=(inherit)
  2a1 : simulink/Math Operations/MinMax Running Resettable  Description=2a  Function=max  vinit=0
  Pulse Generator3 : DiscretePulseGenerator  PulseType=Time based  Period=20  PhaseDelay=23.7
  SW Q_AV : Outport  VectorParamsAs1DForOutWhenUnconnected=off
  wires:
  Pulse Generator3/1 -> 2a1/2
  ? -> 2a1/1
  Outport/1 -> SW Q_AV/1  "SW"

== system Michaels_CVModel_fast8/Stroke Work Calcs/Stroke Work Q_MR/MR Stroke Work Action ==
  PLV : Inport
  QMR : Inport  Port=2
  MRreg : Inport  Port=3
  Action Port : ActionPort  InitializeStates=reset  ActionPortLabel=if(u1 == 1)
  Integrator1 : Integrator  ExternalReset=rising  ZeroCross=off
  Product : Product
  Outport : Outport
  wires:
  PLV/1 -> Product/1
  QMR/1 -> Product/2
  Product/1 -> Integrator1/1
  Integrator1/1 -> Outport/1
  MRreg/1 -> Integrator1/2

== system Michaels_CVModel_fast8/Stroke Work Calcs/Stroke Work Q_MR/Triggered Subsystem1 ==
  Inport : Inport
  Trigger : TriggerPort  TriggerType=falling  VariantControl=(inherit)
  RSW_ Q : Outport  VectorParamsAs1DForOutWhenUnconnected=off
  wires:
  Inport/1 -> RSW_ Q/1  "SW"

== system Michaels_CVModel_fast8/Stroke Work Calcs/Total Stroke Work LV/Triggered Subsystem ==
  In1 : Inport
  In2 : Inport  Port=2
  Trigger : TriggerPort  VariantControl=(inherit)
  Out1 : Outport  VectorParamsAs1DForOutWhenUnconnected=off
  Out2 : Outport  Port=2  VectorParamsAs1DForOutWhenUnconnected=off
  wires:
  In2/1 -> Out2/1  "SW"
  In1/1 -> Out1/1  "Energy"

== system Michaels_CVModel_fast8/ev/Activation - Atria/Action 1 - Sin Squared ==
  In1 : Inport
  Action Port : ActionPort  ActionPortLabel=if(u1 == 1)
  Demux : Demux  Outputs=3
  Gain : Gain  Gain=pi()
  Gain1 : Gain  Gain=2
  Math Function : Math  Operator=square  SignedPower=on  SaturateOnIntegerOverflow=on
  Product18 : Product  Inputs=*/  InputSameDT=on  RndMeth=Zero  SaturateOnIntegerOverflow=on  OutDataTypeStr=Inherit: Same as first input
  Sum3 : Sum  Inputs=+-  InputSameDT=on  SaturateOnIntegerOverflow=on  OutDataTypeStr=Inherit: Same as first input
  Trigonometric Function : Trigonometry
  Out1 : Outport
  wires:
  In1/1 -> Demux/1
  Demux/1 -> Sum3/1  "t"
  Demux/2 -> Sum3/2  "tsh_v"
  Sum3/1 -> Gain/1
  Gain/1 -> Product18/1
  Demux/3 -> Gain1/1
  Gain1/1 -> Product18/2
  Product18/1 -> Trigonometric Function/1
  Trigonometric Function/1 -> Math Function/1
  Math Function/1 -> Out1/1

== system Michaels_CVModel_fast8/ev/Activation - Atria/Action 2 - cos Squared1 ==
  In1 : Inport
  Action Port : ActionPort  ActionPortLabel=elseif(u2 == 1)
  Demux : Demux
  Gain : Gain  Gain=pi()
  Gain1 : Gain  Gain=2
  Math Function : Math  Operator=square  SignedPower=on  SaturateOnIntegerOverflow=on
  Product18 : Product  Inputs=*/  InputSameDT=on  RndMeth=Zero  SaturateOnIntegerOverflow=on  OutDataTypeStr=Inherit: Same as first input
  Sum1 : Sum  Inputs=+-  InputSameDT=on  SaturateOnIntegerOverflow=on  OutDataTypeStr=Inherit: Same as first input
  Sum3 : Sum  Inputs=+--  InputSameDT=on  SaturateOnIntegerOverflow=on  OutDataTypeStr=Inherit: Same as first input
  Trigonometric Function : Trigonometry  Operator=cos
  Out1 : Outport
  wires:
  In1/1 -> Demux/1
  Demux/1 -> Sum3/1  "t"
  Demux/2 -> Sum3/2  "tsh_v"
  Sum3/1 -> Gain/1
  Gain/1 -> Product18/1
  Gain1/1 -> Product18/2
  Product18/1 -> Trigonometric Function/1
  Trigonometric Function/1 -> Math Function/1
  Math Function/1 -> Out1/1
  Demux/3 -> Sum3/3, Sum1/2  "tr"
  Sum1/1 -> Gain1/1
  Demux/4 -> Sum1/1

== system Michaels_CVModel_fast8/ev/Activation - Atria/Condition 1 ==
  note: Condition 1 - Start of Systole
  Logical Operator : Logic  AllPortsSameDT=off  OutDataTypeStr=boolean
  Relational Operator : RelationalOperator  OutDataTypeStr=boolean  RndMeth=Nearest
  Relational Operator1 : RelationalOperator  Operator=<  OutDataTypeStr=boolean  RndMeth=Nearest
  Sum4 : Sum  InputSameDT=on  SaturateOnIntegerOverflow=on  OutDataTypeStr=Inherit: Same as first input
  Out1 : Outport
  wires:
  [t] -> Relational Operator/1
  [Tsh_a] -> Relational Operator/2
  [t] -> Relational Operator1/1
  [Tsh_a] -> Sum4/1
  [Tr_A] -> Sum4/2
  Sum4/1 -> Relational Operator1/2
  Relational Operator/1 -> Logical Operator/1
  Relational Operator1/1 -> Logical Operator/2
  Logical Operator/1 -> Out1/1

== system Michaels_CVModel_fast8/ev/Activation - Atria/Condition 2 ==
  note: Condition 2 - End of Systole
  Logical Operator1 : Logic  AllPortsSameDT=off  OutDataTypeStr=boolean
  Relational Operator2 : RelationalOperator  OutDataTypeStr=boolean  RndMeth=Nearest
  Relational Operator3 : RelationalOperator  Operator=<  OutDataTypeStr=boolean  RndMeth=Nearest
  Sum5 : Sum  InputSameDT=on  SaturateOnIntegerOverflow=on  OutDataTypeStr=Inherit: Same as first input
  Sum6 : Sum  InputSameDT=on  SaturateOnIntegerOverflow=on  OutDataTypeStr=Inherit: Same as first input
  Out1 : Outport
  wires:
  [t] -> Relational Operator2/1
  [t] -> Relational Operator3/1
  [Tsh_a] -> Sum5/1
  [Tr_A] -> Sum5/2
  Relational Operator2/1 -> Logical Operator1/1
  Relational Operator3/1 -> Logical Operator1/2
  Sum5/1 -> Relational Operator2/2
  [Tsh_a] -> Sum6/1
  [TsysA] -> Sum6/2
  Sum6/1 -> Relational Operator3/2
  Logical Operator1/1 -> Out1/1

== system Michaels_CVModel_fast8/ev/Activation - Atria/Else - 0 ==
  Action Port : ActionPort  ActionPortLabel=else
  venk3 : Constant  Value=0
  Out1 : Outport
  wires:
  venk3/1 -> Out1/1

== system Michaels_CVModel_fast8/ev/Activation - Ventricle/Action 1 - Sin Squared ==
  In1 : Inport
  Action Port : ActionPort  ActionPortLabel=if(u1 == 1)
  Demux : Demux  Outputs=3
  Gain : Gain  Gain=pi()
  Gain1 : Gain  Gain=2
  Math Function : Math  Operator=square  SignedPower=on  SaturateOnIntegerOverflow=on
  Product18 : Product  Inputs=*/  InputSameDT=on  RndMeth=Zero  SaturateOnIntegerOverflow=on  OutDataTypeStr=Inherit: Same as first input
  Sum3 : Sum  Inputs=+-  InputSameDT=on  SaturateOnIntegerOverflow=on  OutDataTypeStr=Inherit: Same as first input
  Trigonometric Function : Trigonometry
  Out1 : Outport
  wires:
  In1/1 -> Demux/1
  Demux/1 -> Sum3/1  "t"
  Demux/2 -> Sum3/2  "tsh_v"
  Sum3/1 -> Gain/1
  Gain/1 -> Product18/1
  Demux/3 -> Gain1/1
  Gain1/1 -> Product18/2
  Product18/1 -> Trigonometric Function/1
  Trigonometric Function/1 -> Math Function/1
  Math Function/1 -> Out1/1

== system Michaels_CVModel_fast8/ev/Activation - Ventricle/Action 2 - cos Squared1 ==
  In1 : Inport
  Action Port : ActionPort  ActionPortLabel=elseif(u2 == 1)
  Demux : Demux
  Gain : Gain  Gain=pi()
  Gain1 : Gain  Gain=2
  Math Function : Math  Operator=square  SignedPower=on  SaturateOnIntegerOverflow=on
  Product18 : Product  Inputs=*/  InputSameDT=on  RndMeth=Zero  SaturateOnIntegerOverflow=on  OutDataTypeStr=Inherit: Same as first input
  Sum1 : Sum  Inputs=+-  InputSameDT=on  SaturateOnIntegerOverflow=on  OutDataTypeStr=Inherit: Same as first input
  Sum3 : Sum  Inputs=+--  InputSameDT=on  SaturateOnIntegerOverflow=on  OutDataTypeStr=Inherit: Same as first input
  Trigonometric Function : Trigonometry  Operator=cos
  Out1 : Outport
  wires:
  In1/1 -> Demux/1
  Demux/1 -> Sum3/1  "t"
  Demux/2 -> Sum3/2  "tsh_v"
  Sum3/1 -> Gain/1
  Gain/1 -> Product18/1
  Gain1/1 -> Product18/2
  Product18/1 -> Trigonometric Function/1
  Trigonometric Function/1 -> Math Function/1
  Math Function/1 -> Out1/1
  Demux/3 -> Sum3/3, Sum1/2  "tr"
  Sum1/1 -> Gain1/1
  Demux/4 -> Sum1/1

== system Michaels_CVModel_fast8/ev/Activation - Ventricle/Condition 1 ==
  note: Condition 1 - Start of Systole
  Logical Operator : Logic  AllPortsSameDT=off  OutDataTypeStr=boolean
  Relational Operator : RelationalOperator  OutDataTypeStr=boolean  RndMeth=Nearest
  Relational Operator1 : RelationalOperator  Operator=<  OutDataTypeStr=boolean  RndMeth=Nearest
  Sum4 : Sum  InputSameDT=on  SaturateOnIntegerOverflow=on  OutDataTypeStr=Inherit: Same as first input
  Out1 : Outport
  wires:
  [t] -> Relational Operator/1
  [Tsh_v] -> Relational Operator/2
  [t] -> Relational Operator1/1
  [Tsh_v] -> Sum4/1
  [Tr_V] -> Sum4/2
  Sum4/1 -> Relational Operator1/2
  Relational Operator/1 -> Logical Operator/1
  Relational Operator1/1 -> Logical Operator/2
  Logical Operator/1 -> Out1/1

== system Michaels_CVModel_fast8/ev/Activation - Ventricle/Condition 2 ==
  note: Condition 2 - End of Systole
  Logical Operator1 : Logic  AllPortsSameDT=off  OutDataTypeStr=boolean
  Relational Operator2 : RelationalOperator  OutDataTypeStr=boolean  RndMeth=Nearest
  Relational Operator3 : RelationalOperator  Operator=<  OutDataTypeStr=boolean  RndMeth=Nearest
  Sum5 : Sum  InputSameDT=on  SaturateOnIntegerOverflow=on  OutDataTypeStr=Inherit: Same as first input
  Sum6 : Sum  InputSameDT=on  SaturateOnIntegerOverflow=on  OutDataTypeStr=Inherit: Same as first input
  Out1 : Outport
  wires:
  [t] -> Relational Operator2/1
  [t] -> Relational Operator3/1
  [Tsh_v] -> Sum5/1
  [Tr_V] -> Sum5/2
  Relational Operator2/1 -> Logical Operator1/1
  Relational Operator3/1 -> Logical Operator1/2
  Sum5/1 -> Relational Operator2/2
  [Tsh_v] -> Sum6/1
  [TsysV] -> Sum6/2
  Sum6/1 -> Relational Operator3/2
  Logical Operator1/1 -> Out1/1

== system Michaels_CVModel_fast8/ev/Activation - Ventricle/Else - 0 ==
  Action Port : ActionPort  ActionPortLabel=else
  venk3 : Constant  Value=0
  Out1 : Outport
  wires:
  venk3/1 -> Out1/1

== system Michaels_CVModel_fast8/ev/Activation - Ventricle_half/Action 1 - Sin Squared ==
  In1 : Inport
  Action Port : ActionPort  ActionPortLabel=if(u1 == 1)
  Demux : Demux  Outputs=3
  For a zero ouput : Gain  Gain=0
  Gain : Gain  Gain=pi()
  Gain1 : Gain  Gain=2
  Math Function : Math  Operator=square  SignedPower=on  SaturateOnIntegerOverflow=on
  Product18 : Product  Inputs=*/  InputSameDT=on  RndMeth=Zero  SaturateOnIntegerOverflow=on  OutDataTypeStr=Inherit: Same as first input
  Sum3 : Sum  Inputs=+-  InputSameDT=on  SaturateOnIntegerOverflow=on  OutDataTypeStr=Inherit: Same as first input
  Trigonometric Function : Trigonometry
  Out1 : Outport
  wires:
  In1/1 -> Demux/1
  Demux/1 -> Sum3/1  "t"
  Demux/2 -> Sum3/2  "tsh_v"
  Sum3/1 -> Gain/1
  Gain/1 -> Product18/1
  Demux/3 -> Gain1/1
  Gain1/1 -> Product18/2
  Product18/1 -> Trigonometric Function/1
  Trigonometric Function/1 -> Math Function/1
  Math Function/1 -> For a zero ouput/1
  For a zero ouput/1 -> Out1/1

== system Michaels_CVModel_fast8/ev/Activation - Ventricle_half/Action 2 - cos Squared1 ==
  In1 : Inport
  Action Port : ActionPort  ActionPortLabel=elseif(u2 == 1)
  Demux : Demux
  Gain : Gain  Gain=pi()
  Gain1 : Gain  Gain=2
  Math Function : Math  Operator=square  SignedPower=on  SaturateOnIntegerOverflow=on
  Product18 : Product  Inputs=*/  InputSameDT=on  RndMeth=Zero  SaturateOnIntegerOverflow=on  OutDataTypeStr=Inherit: Same as first input
  Sum1 : Sum  Inputs=+-  InputSameDT=on  SaturateOnIntegerOverflow=on  OutDataTypeStr=Inherit: Same as first input
  Sum3 : Sum  Inputs=+--  InputSameDT=on  SaturateOnIntegerOverflow=on  OutDataTypeStr=Inherit: Same as first input
  Trigonometric Function : Trigonometry  Operator=cos
  Out1 : Outport
  wires:
  In1/1 -> Demux/1
  Demux/1 -> Sum3/1  "t"
  Demux/2 -> Sum3/2  "tsh_v"
  Sum3/1 -> Gain/1
  Gain/1 -> Product18/1
  Gain1/1 -> Product18/2
  Product18/1 -> Trigonometric Function/1
  Trigonometric Function/1 -> Math Function/1
  Math Function/1 -> Out1/1
  Demux/3 -> Sum3/3, Sum1/2  "tr"
  Sum1/1 -> Gain1/1
  Demux/4 -> Sum1/1

== system Michaels_CVModel_fast8/ev/Activation - Ventricle_half/Condition 1 ==
  note: Condition 1 - Start of Systole
  Logical Operator : Logic  AllPortsSameDT=off  OutDataTypeStr=boolean
  Relational Operator : RelationalOperator  OutDataTypeStr=boolean  RndMeth=Nearest
  Relational Operator1 : RelationalOperator  Operator=<  OutDataTypeStr=boolean  RndMeth=Nearest
  Sum4 : Sum  InputSameDT=on  SaturateOnIntegerOverflow=on  OutDataTypeStr=Inherit: Same as first input
  Out1 : Outport
  wires:
  [t] -> Relational Operator/1
  [Tsh_v] -> Relational Operator/2
  [t] -> Relational Operator1/1
  [Tsh_v] -> Sum4/1
  [Tr_V] -> Sum4/2
  Sum4/1 -> Relational Operator1/2
  Relational Operator/1 -> Logical Operator/1
  Relational Operator1/1 -> Logical Operator/2
  Logical Operator/1 -> Out1/1

== system Michaels_CVModel_fast8/ev/Activation - Ventricle_half/Condition 2 ==
  note: Condition 2 - End of Systole
  Logical Operator1 : Logic  AllPortsSameDT=off  OutDataTypeStr=boolean
  Relational Operator2 : RelationalOperator  OutDataTypeStr=boolean  RndMeth=Nearest
  Relational Operator3 : RelationalOperator  Operator=<  OutDataTypeStr=boolean  RndMeth=Nearest
  Sum5 : Sum  InputSameDT=on  SaturateOnIntegerOverflow=on  OutDataTypeStr=Inherit: Same as first input
  Sum6 : Sum  InputSameDT=on  SaturateOnIntegerOverflow=on  OutDataTypeStr=Inherit: Same as first input
  Out1 : Outport
  wires:
  [t] -> Relational Operator2/1
  [t] -> Relational Operator3/1
  [Tsh_v] -> Sum5/1
  [Tr_V] -> Sum5/2
  Relational Operator2/1 -> Logical Operator1/1
  Relational Operator3/1 -> Logical Operator1/2
  Sum5/1 -> Relational Operator2/2
  [Tsh_v] -> Sum6/1
  [TsysV] -> Sum6/2
  Sum6/1 -> Relational Operator3/2
  Logical Operator1/1 -> Out1/1

== system Michaels_CVModel_fast8/ev/Activation - Ventricle_half/Else - 0 ==
  Action Port : ActionPort  ActionPortLabel=else
  venk3 : Constant  Value=0
  Out1 : Outport
  wires:
  venk3/1 -> Out1/1

== matlab function Michaels_CVModel_fast8/Baroreflex/Baroreflex Lu/Fvaso ==
  data: Nvaso input; Fvaso output
function Fvaso = fcn(Nvaso)
%#eml

a=0.3;
b=0.7;
Nx0=110;
txs=0.04;
Fvaso=a+(b/(exp(txs*(Nvaso-Nx0))+1));

== matlab function Michaels_CVModel_fast8/Baroreflex/Baroreflex Lu/FhrV ==
  data: Nhrv input; Fhrv output
function Fhrv = fcn(Nhrv)
%#codegen

a=0;
b=1;
Nx0=110;
txs=-0.04;
Fhrv=a+(b/(exp(txs*(Nhrv-Nx0))+1));

== matlab function Michaels_CVModel_fast8/Baroreflex/Baroreflex Lu/FhrS ==
  data: Nhrs input; Fhrs output
function Fhrs = fcn(Nhrs)
%#eml

a=0.3;
b=0.7;
Nx0=100;
txs=0.09;
Fhrs=a+(b/(exp(txs*(Nhrs-Nx0))+1));

== matlab function Michaels_CVModel_fast8/Baroreflex/Baroreflex Lu/Fcon ==
  data: Nvaso input; Fvaso output
function Fvaso = fcn(Nvaso)
%#eml

a=0.3;
b=0.7;
Nx0=110;
txs=0.04;
Fvaso=a+(b/(exp(txs*(Nvaso-Nx0))+1));

== matlab function Michaels_CVModel_fast8/Baroreflex/Baroreflex Lu/Contractility Function ==
  data: Fcon input; aFcon output; amin input; Ka input
function aFcon = fcn(Fcon, amin, Ka)
%This is the function used to calculate Rsa from the equation provided
%by Lu
% amin = -2;
% Ka = 5;

aFcon = amin + Ka*Fcon;

== matlab function Michaels_CVModel_fast8/Key Outputs/00 Date & Time/MATLAB Function ==
  data: D output; u input
function D  = fcn(u)
   eml.extrinsic('now');
   eml.extrinsic('datenum');
   Y = 0;
   M = 0;
   D = 0;
   H = 0;
   MN = 0;
   S = 0;
   [D] = datenum(now);
end

== matlab function Michaels_CVModel_fast8/Baroreflex/Baroreflex Lu/HR transfer Function ==
  data: Fhrv input; HR output; Fhrs input
function HR = fcn(Fhrv,Fhrs)
%This is the function provided by Lu using normalized
%vagal and sympathetic frequencies to calculate heart rate
h1=35; % originally 35
h2=140;
h3=40;
h4=32;
h5=10;
h6=20; %originally 20
HR=h1+h2*Fhrs-h3*Fhrs^2-h4*Fhrv+h5*Fhrv^2-h6*Fhrv*Fhrs;

== matlab function Michaels_CVModel_fast8/Baroreflex/Baroreflex Lu/Rsa Trans Fn ==
  data: Fvaso input; Rsa output; Vsa input
function Rsa = fcn(Fvaso, Vsa)
%This is the function used to calculate Rsa from the equation provided
%by Lu
Kr=0.04;
Vsamax=250;
Vsa_temp=210;
Rsa=Kr*exp(4*Fvaso)+0*Kr*((Vsamax/Vsa_temp)^2);
